simulink model "positionexample2class"  (R2022a)
settings: Solver=ode3  StartTime=0.0  StopTime=30  FixedStep=ts  RelTol=1e-3  EnableMultiTasking=on
undefined symbols (not defined in the file): motor_rev, ts
libraries: raspberrypiBasiclib x4, slpidlib x1, dspsrcs4 x1
settings Model: ExtModeTrigDuration=2  Creator=tsuga  LastModifiedBy=admin
settings SolverCC: PositivePriorityOrder=on  AutoInsertRateTranBlk=on
settings DataIOCC: SaveOutput=off  SignalLogging=off  DSMLogging=off  SaveTime=off  ReturnWorkspaceOutputs=off
settings OptimizationCC: EnhancedBackFolding=on  PassReuseOutputArgsAs=Individual arguments  ZeroExternalMemoryAtStartup=off  ZeroInternalMemoryAtStartup=off  MaxStackSize=64  OptimizeBlockOrder=speed  DifferentSizesBufferReuse=on  EfficientTunableParamExpr=on
settings DebuggingCC: ParameterTunabilityLossMsg=error  UnconnectedInputMsg=warning  UnconnectedOutputMsg=warning  UnconnectedLineMsg=warning
settings HardwareCC: ProdBitPerPointer=32  ProdBitPerSizeT=32  ProdBitPerPtrDiffT=32  ProdLargestAtomicInteger=Long  ProdLargestAtomicFloat=Double  ProdWordSize=32  ProdLongLongMode=on  ProdHWDeviceType=ARM Compatible->ARM Cortex
settings RTWCC: SystemTargetFile=ert.tlc  HardwareBoard=Raspberry Pi  TLCOptions="-aInlineSetEventsForThisBaseRateFcn=TLC_FALSE -aSuppressMultiTaskScheduler=TLC_FALSE  -aRateBasedStepFcn=0"  TemplateMakefile=ert_default_tmf  Toolchain=GNU GCC Embedded Linux  BuildConfiguration=Faster Runs  DLArmComputeVersion=19.05
settings CodeAppCC: ForceParamTrailComments=on  IgnoreCustomStorageClasses=off  OperatorAnnotations=on  SimulinkDataObjDesc=on  SFDataObjDesc=on  InsertBlockDesc=on
settings ERTTargetCC: SupportContinuousTime=on  SupportNonInlinedSFcns=on  SupportVariableSizeSignals=on

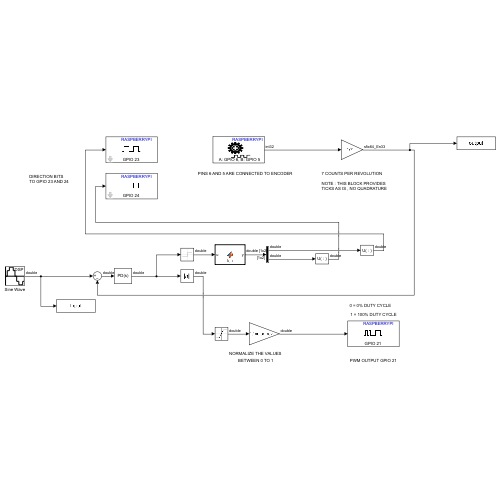
[thumbnail: Simulink's stored preview of the top-level diagram]
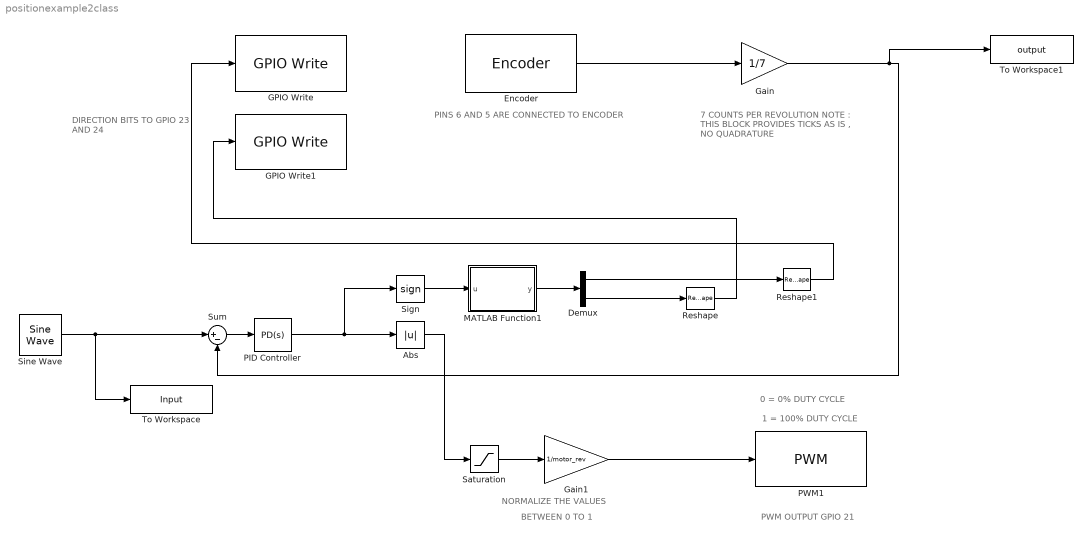
== system positionexample2class ==
  note: 1 = 100% DUTY CYCLE
  note: 0 = 0% DUTY CYCLE
  note: BETWEEN 0 TO 1
  note: NORMALIZE THE VALUES
  note: PWM OUTPUT GPIO 21
  note: DIRECTION BITS
      | TO GPIO 23 AND 24
  note: 7 COUNTS PER REVOLUTION
      |
      | NOTE : THIS BLOCK PROVIDES
      | TICKS AS IS , NO QUADRATURE
  note: PINS 6 AND 5 ARE CONNECTED TO ENCODER
  Abs : Abs  SaturateOnIntegerOverflow=off
  Demux : Demux  Outputs=2
  Encoder : raspberrypiBasiclib/Encoder  BoardProperty=Pi 4 Model B  InputA=GPIO 6  InputB=GPIO 5  Mode=No reset  SampleTime=ts
      settings: SourceProductBaseCode=RASPPI
  GPIO Write : raspberrypiBasiclib/GPIO Write  board=Model B+  gpio=23  direction=Output  blockPlatform=Raspberry Pi
      settings: SourceProductBaseCode=RASPPI
  GPIO Write1 : raspberrypiBasiclib/GPIO Write  board=Model B+  gpio=24  direction=Output  blockPlatform=Raspberry Pi
      settings: SourceProductBaseCode=RASPPI
  Gain : Gain  Gain=1/7
  Gain1 : Gain  Gain=1/motor_rev
  MATLAB Function1 : MATLAB Function  TreatAsAtomicUnit=on
  PID Controller : slpidlib/PID Controller  Controller=PD  Form=Parallel  TimeDomain=Continuous-time  UseExternalTs=off  SampleTime=-1  IntegratorMethod=Forward Euler  FilterMethod=Forward Euler  ControllerParametersSource=internal  P=15  I=1  UseKiTs=off  D=0.5  N=100  UseFilter=on  TunerSelectOption=Frequency Response Based  InitialConditionSource=internal  InitialConditionForIntegrator=0  InitialConditionForFilter=0  DifferentiatorICPrevScaledInput=0  ExternalReset=none  TrackingMode=off  Kt=1  LimitOutput=off  SatLimitsSource=internal  UpperSaturationLimit=inf  LowerSaturationLimit=-inf  LinearizeAsGain=on  AntiWindupMode=none  Kb=1  POutMin=[]  POutMax=[]  IOutMin=[]  IOutMax=[]  DOutMin=[]  DOutMax=[]  NOutMin=[]  NOutMax=[]  SumOutMin=[]  SumOutMax=[]  SaturationOutMin=[]  SaturationOutMax=[]  PParamMin=[]  PParamMax=[]  IParamMin=[]  IParamMax=[]  DParamMin=[]  DParamMax=[]  NParamMin=[]  NParamMax=[]  KbParamMin=[]  KbParamMax=[]  KtParamMin=[]  KtParamMax=[]  KbOutMin=[]  KbOutMax=[]  KtOutMin=[]  KtOutMax=[]  IntegratorOutMin=[]  IntegratorOutMax=[]  FilterOutMin=[]  FilterOutMax=[]  SumI1OutMin=[]  SumI1OutMax=[]  SumI2OutMin=[]  SumI2OutMax=[]  SumI3OutMin=[]  SumI3OutMax=[]  SumI4OutMin=[]  SumI4OutMax=[]  SumDOutMin=[]  SumDOutMax=[]  DifferentiatorOutMin=[]  DifferentiatorOutMax=[]  FilterDiffOutCoefMin=[]  FilterDiffOutCoefMax=[]  ReciprocalOutMin=[]  ReciprocalOutMax=[]  SumDenOutMin=[]  SumDenOutMax=[]  SumNumOutMin=[]  SumNumOutMax=[]  DivideOutMin=[]  DivideOutMax=[]  UdiffTsProdOutMin=[]  UdiffTsProdOutMax=[]  NTsProdOutMin=[]  NTsProdOutMax=[]  UintegralTsProdOutMin=[]  UintegralTsProdOutMax=[]  UngainTsProdOutMin=[]  UngainTsProdOutMax=[]  IntegratorContinuousStateAttributes=''  IntegratorStateMustResolveToSignalObject=off  IntegratorRTWStateStorageClass=Auto  FilterContinuousStateAttributes=''  FilterStateMustResolveToSignalObject=off  FilterRTWStateStorageClass=Auto  ParallelPVariant=InternalParameters  IdealPVariant=Disabled  IVariant=Disabled  DVariant=InternalParameters  IntegratorVariant=Disabled  SatVariant=Disabled  AWVariant=Disabled  PCopyVariant=Disabled  TRVariant=Disabled  FdbkBlocksVariant=Forward  IdealPFdbkVariant=Disabled  SatFdbkVariant=Disabled  DerivativeFilterVariant=ContFilter  NVariant=InternalParameters  NCopyVariant=Disabled  FilterICVariant=InternalICsFilter  IntegratorICVariant=Disabled  ExternalResetVariant=Disabled  TRSumVariant=Passthrough  SumFdbkVariant=Disabled  SumVariant=Sum_PD  TsampFilterVariant=InternalTs  TsampNgainVariant=Passthrough  TsampIntegralVariant=Disabled_SignalSpec  ExternalSaturationOutDataTypeStr=Inherit: Same as second input  aMode=0
  PWM1 : raspberrypiBasiclib/PWM  board=Pi 2 Model B  Pin_=21  Frequency=500  blockPlatform=Raspberry Pi
      settings: SourceProductBaseCode=RASPPI
  Reshape : Reshape
  Reshape1 : Reshape
  Saturation : Saturate  UpperLimit=motor_rev  LowerLimit=0
  Sign : Signum
  Sine Wave : dspsrcs4/Sine Wave  Amplitude=motor_rev  Frequency=0.2  Phase=0  SampleMode=Discrete  OutComplex=Real  CompMethod=Trigonometric fcn  TableSize=Speed  SampleTime=ts  SamplesPerFrame=1  ResetState=Restart at time zero  OutputFrames=off  dataType=double  wordLen=16  udDataType=sfix(16)  fracBitsMode=Best precision  numFracBits=15  OutDataTypeStr=double  LastOutDataTypeStr=double
  Sum : Sum  Inputs=|+-
  To Workspace : ToWorkspace  VariableName=Input  SampleTime=-1
      settings: Save2DSignal=2-D array (concatenate along first dimension)
  To Workspace1 : ToWorkspace  VariableName=output  SampleTime=-1
      settings: Save2DSignal=2-D array (concatenate along first dimension)
  wires:
  Abs/1 -> Saturation/1
  Gain1/1 -> PWM1/1
  Reshape/1 -> GPIO Write1/1
  Reshape1/1 -> GPIO Write/1
  Demux/1 -> Reshape1/1
  Demux/2 -> Reshape/1
  Sine Wave/1 -> Sum/1, To Workspace/1
  Sign/1 -> MATLAB Function1/1(u)
  MATLAB Function1/1(y) -> Demux/1
  Gain/1 -> Sum/2, To Workspace1/1
  Encoder/1 -> Gain/1
  Saturation/1 -> Gain1/1
  PID Controller/1 -> Sign/1, Abs/1
  Sum/1 -> PID Controller/1

== matlab function positionexample2class/MATLAB Function1 ==
  data: u input; y output
function y = fcn(u)
%#codegen

% xx = typecast(u,'single');
% y=xx(1);

y=zeros(1,2);  % this method worked

if u > 0
    y(1) = 1;
    y(2) = 0;
elseif u < 0
    y(1) = 0;
    y(2) = 1;
end
